simulink model "IT1_FPID_Controller"  (R2018b)
settings: Solver=VariableStepAuto  StartTime=0.0  StopTime=10.0  RelTol=1e-3
values from neighbouring files (symbols this model uses):
  K = 1    [runControlSystemExample_fis1.m]
  Ka = 0.077    [runControlSystemExample_fis1.m]
  Kb = 7.336    [runControlSystemExample_fis1.m]
  Kd = 0.5141    [runControlSystemExample_fis1.m]
  Ke = 1    [runControlSystemExample_fis1.m]
  L = 0.3    [runControlSystemExample_fis1.m]
  T = 1.1    [runControlSystemExample_fis1.m]
libraries: fuzblock x1
settings Model: Creator=Ivan Milin  LastModifiedBy=Ivan Milin

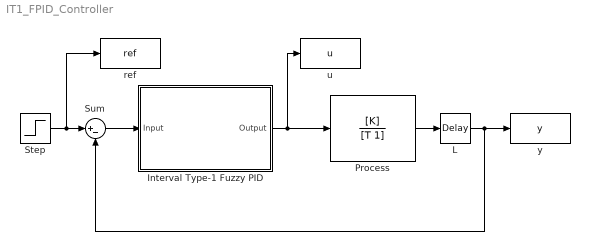
== system IT1_FPID_Controller ==
  Interval Type-1 Fuzzy PID : Subsystem
  L : TransportDelay  DelayTime=L
  Process : TransferFcn  Numerator=[K]  Denominator=[T 1]
  Step : Step  SampleTime=0
  Sum : Sum  Inputs=|+-
  ref : ToWorkspace  VariableName=ref  SaveFormat=Structure With Time  SampleTime=-1
  u : ToWorkspace  VariableName=u  SaveFormat=Structure With Time  SampleTime=-1
  y : ToWorkspace  VariableName=y  SaveFormat=Structure With Time  SampleTime=-1
  wires:
  L/1 -> Sum/2, y/1
  Process/1 -> L/1
  Sum/1 -> Interval Type-1 Fuzzy PID/1(Input)
  Step/1 -> ref/1, Sum/1
  Interval Type-1 Fuzzy PID/1(Output) -> u/1, Process/1

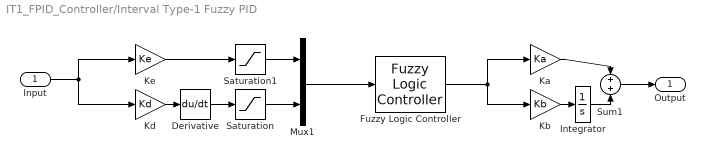
== system IT1_FPID_Controller/Interval Type-1 Fuzzy PID ==
  Input : Inport
  Derivative : Derivative
  Fuzzy Logic Controller : fuzblock/Fuzzy Logic  Controller  FIS='zadatak2b.fis'  OutputSampleNumber=101  DataType=double  FuzzifiedInputs=off  RuleFiringStrengths=off  RuleOutputs=off  AggregatedOutputs=off  SimulateUsing=Interpreted execution  OutOfRangeInputValueMessage=warning  NoRuleFiredMessage=warning  EmptyOutputFuzzySetMessage=warning
  Integrator : Integrator
  Ka : Gain  Gain=Ka
  Kb : Gain  Gain=Kb
  Kd : Gain  Gain=Kd
  Ke : Gain  Gain=Ke
  Mux1 : Mux  Inputs=2
  Saturation : Saturate  UpperLimit=1  LowerLimit=-1
  Saturation1 : Saturate  UpperLimit=1  LowerLimit=-1
  Sum1 : Sum
  Output : Outport
  wires:
  Saturation1/1 -> Mux1/1
  Saturation/1 -> Mux1/2
  Derivative/1 -> Saturation/1
  Kd/1 -> Derivative/1
  Ke/1 -> Saturation1/1
  Input/1 -> Kd/1, Ke/1
  Fuzzy Logic Controller/1 -> Kb/1, Ka/1
  Kb/1 -> Integrator/1
  Integrator/1 -> Sum1/2
  Ka/1 -> Sum1/1
  Sum1/1 -> Output/1
  Mux1/1 -> Fuzzy Logic Controller/1
